simulink model "validation_gate_test"  (Simulink 7.6)
settings: Solver=FixedStepDiscrete  StartTime=0.0  StopTime=0  RelTol=1e-3
undefined symbols (not defined in the file or in its folder): Buoy_Count_Max, Buoy_Count_Min, Buoy_Max_Eccentricity, Buoy_Max_Extent, Buoy_Min_Eccentricity, Buoy_Min_Extent, Hedge_Hue, Iter_Segment_Thresh, Rec, SDTV, strel
libraries: vipconversions x6, vipgeotforms x3, simulink x2, viptextngfix x2, viptransforms x2, vipmorphops x1, vipanalysis x1
(part 1 of 2)
settings Model: Creator=Thing 1  LastModifiedBy=auvt

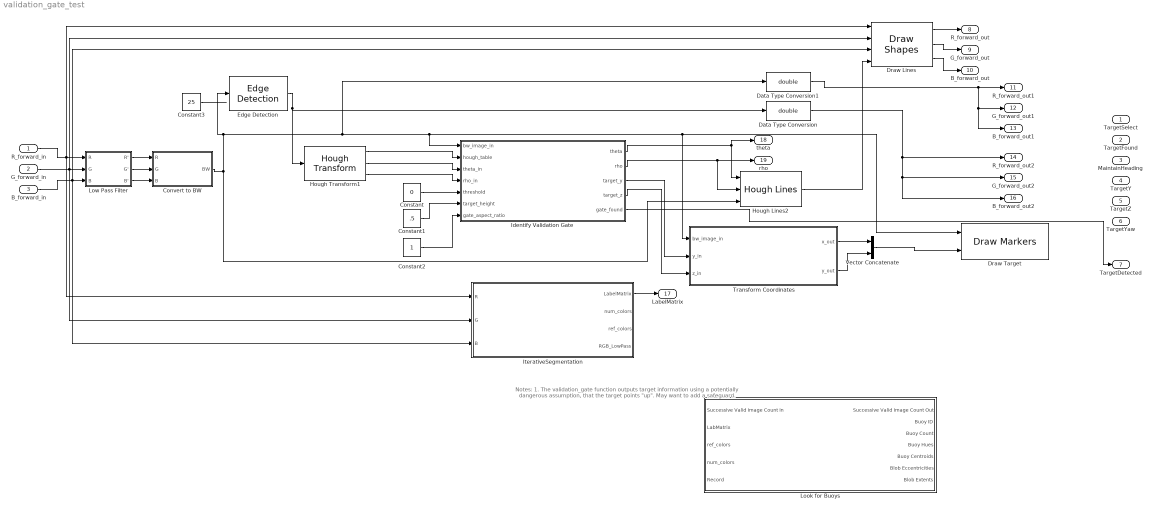
== system validation_gate_test ==
  note: Notes:
      | 1. The validation_gate function outputs target
      | information using a potentially dangerous
      | assumption, that the target points "up". May
      | want to add a safeguard.
  R_forward_in : Inport  PortDimensions=[120 160]
  G_forward_in : Inport  Port=2  PortDimensions=[120 160]
  B_forward_in : Inport  Port=3  PortDimensions=[120 160]
  Constant : Constant  Value=0  SampleTime=-1
  Constant1 : Constant  Value=.5  SampleTime=-1
  Constant2 : Constant  SampleTime=-1
  Constant3 : Constant  Value=25  SampleTime=-1
  Convert to BW : Subsystem
  Data Type Conversion : DataTypeConversion  OutDataTypeStr=double
  Data Type Conversion1 : DataTypeConversion  OutDataTypeStr=double
  Draw Lines : viptextngfix/Draw Shapes  DialogController=vipDDGCreate  DialogControllerArgs=DataTag3  shape=Lines  fill=off  fillClrSource=Specify via dialog  display=User-specified value  intensity=200  color=[.8 .8 .8]  opacity=0.6  viewport=Entire image  antialiasing=off  inType=Obsolete  imagePorts=Separate color signals  prodOutputMode=Binary point scaling  prodOutputWordLength=32  prodOutputFracLength=14  memoryMode=Specify word length  memoryWordLength=16  memoryFracLength=15  roundingMode=Floor  overflowMode=off
  Draw Target : viptextngfix/Draw Markers  DialogController=vipDDGCreate  DialogControllerArgs=DataTag4  shape=X-mark  size=7  fill=off  fillClrSource=Specify via dialog  display=User-specified value  intensity=200  color=0  opacity=0.6  viewport=Entire image  antialiasing=off  inType=Obsolete  imagePorts=One multidimensional signal  prodOutputMode=Binary point scaling  prodOutputWordLength=32  prodOutputFracLength=14  memoryMode=Specify word length  memoryWordLength=16  memoryFracLength=15  roundingMode=Floor  overflowMode=off
  Edge Detection : vipanalysis/Edge Detection  DialogController=vipDDGCreate  DialogControllerArgs=DataTag5  method=Sobel  outputType=Binary image  userDefinedThreshold=off  thresholdSource=Specify via dialog  threshold=20  thresholdTuning=3  edgeThinning=on  threshold_canny=[0.25 0.60]  autoPercent=70  sigma=1  roundingMode=Floor  overflowMode=off
  Hough Lines2 : viptransforms/Hough Lines  DialogController=vipDDGCreate  DialogControllerArgs=DataTag6  sineCompMethod=Trigonometric function  thetaRes=pi/180  firstCoeffMode=Specify word length  firstCoeffWordLength=16  firstCoeffFracLength=15  prodOutputMode=Binary point scaling  prodOutputWordLength=32  prodOutputFracLength=16  roundingMode=Nearest  overflowMode=on
  Hough Transform1 : viptransforms/Hough Transform  DialogController=vipDDGCreate  DialogControllerArgs=DataTag7  theta_res=.5*pi/180  rho_res=1  out_theta_rho=on  outdtmode=double  firstCoeffMode=Binary point scaling  firstCoeffWordLength=16  firstCoeffFracLength=14  secondCoeffMode=Binary point scaling  secondCoeffWordLength=32  secondCoeffFracLength=16  outputMode=Binary point scaling  outputWordLength=16  outputFracLength=0  accumMode=Binary point scaling  accumWordLength=32  accumFracLength=20  prodOutputMode=Binary point scaling  prodOutputWordLength=32  prodOutputFracLength=20  memoryMode=Binary point scaling  memoryWordLength=32  memoryFracLength=16  roundingMode=Nearest  overflowMode=on
  Identify Validation Gate : Stateflow chart  TreatAsAtomicUnit=on  SystemSampleTime=[1/30 0]
  IterativeSegmentation : Subsystem
      settings: UndoDeleteFcn=Stateflow.SLINSF.SimulinkMan.restorePreDeleteFcn  PreDeleteFcn=Stateflow.SLINSF.SimulinkMan.removePreDeleteFcn
  Look for Buoys : Subsystem
      settings: UndoDeleteFcn=Stateflow.SLINSF.SimulinkMan.restorePreDeleteFcn  PreDeleteFcn=Stateflow.SLINSF.SimulinkMan.removePreDeleteFcn
  Low Pass Filter : Subsystem
  Transform Coordinates : Stateflow chart  TreatAsAtomicUnit=on  SystemSampleTime=[1/30 0]
  Vector Concatenate : Concatenate  Mode=Multidimensional array
  TargetSelect : Outport  OutDataTypeStr=double
  TargetFound : Outport  Port=2  OutDataTypeStr=double
  MaintainHeading : Outport  Port=3  OutDataTypeStr=double
  TargetY : Outport  Port=4  OutDataTypeStr=double
  TargetZ : Outport  Port=5  OutDataTypeStr=double
  TargetYaw : Outport  Port=6  OutDataTypeStr=double
  TargetDetected : Outport  Port=7  OutDataTypeStr=double
  R_forward_out : Outport  Port=8  OutDataTypeStr=double
  G_forward_out : Outport  Port=9  OutDataTypeStr=double
  B_forward_out : Outport  Port=10  OutDataTypeStr=double
  R_forward_out1 : Outport  Port=11  OutDataTypeStr=double
  G_forward_out1 : Outport  Port=12  OutDataTypeStr=double
  B_forward_out1 : Outport  Port=13  OutDataTypeStr=double
  R_forward_out2 : Outport  Port=14  OutDataTypeStr=double
  G_forward_out2 : Outport  Port=15  OutDataTypeStr=double
  B_forward_out2 : Outport  Port=16  OutDataTypeStr=double
  LabelMatrix : Outport  Port=17  OutDataTypeStr=double
  theta : Outport  Port=18  OutDataTypeStr=double
  rho : Outport  Port=19  OutDataTypeStr=double
  wires:
  Convert to BW/1(BW) -> Hough Lines2/3, Edge Detection/1, Identify Validation Gate/1(bw_image_in), Transform Coordinates/1(bw_image_in), Draw Target/1, Data Type Conversion1/1
  Hough Transform1/1 -> Identify Validation Gate/2(hough_table)
  Hough Transform1/2 -> Identify Validation Gate/3(theta_in)
  Hough Transform1/3 -> Identify Validation Gate/4(rho_in)
  Edge Detection/1 -> Hough Transform1/1, Data Type Conversion/1
  Constant/1 -> Identify Validation Gate/5(threshold)
  Constant1/1 -> Identify Validation Gate/6(target_height)
  Constant2/1 -> Identify Validation Gate/7(gate_aspect_ratio)
  Identify Validation Gate/1(theta) -> Hough Lines2/1, theta/1
  Identify Validation Gate/2(rho) -> Hough Lines2/2, rho/1
  Identify Validation Gate/3(target_y) -> Transform Coordinates/2(y_in)
  Identify Validation Gate/4(target_z) -> Transform Coordinates/3(z_in)
  Transform Coordinates/1(x_out) -> Vector Concatenate/1
  Transform Coordinates/2(y_out) -> Vector Concatenate/2
  Vector Concatenate/1 -> Draw Target/2
  Identify Validation Gate/5(gate_found) -> TargetDetected/1
  Low Pass Filter/2(G') -> Convert to BW/2(G)
  Low Pass Filter/3(B') -> Convert to BW/3(B)
  G_forward_in/1 -> Low Pass Filter/2(G), IterativeSegmentation/2(G), Draw Lines/2
  B_forward_in/1 -> Low Pass Filter/3(B), IterativeSegmentation/3(B), Draw Lines/3
  Low Pass Filter/1(R') -> Convert to BW/1(R)
  R_forward_in/1 -> Low Pass Filter/1(R), IterativeSegmentation/1(R), Draw Lines/1
  Constant3/1 -> ?
  Data Type Conversion1/1 -> R_forward_out1/1, G_forward_out1/1, B_forward_out1/1
  IterativeSegmentation/1(LabelMatrix) -> LabelMatrix/1
  Data Type Conversion/1 -> R_forward_out2/1, G_forward_out2/1, B_forward_out2/1
  Draw Lines/1 -> R_forward_out/1
  Draw Lines/2 -> G_forward_out/1
  Draw Lines/3 -> B_forward_out/1
  Hough Lines2/1 -> Draw Lines/4

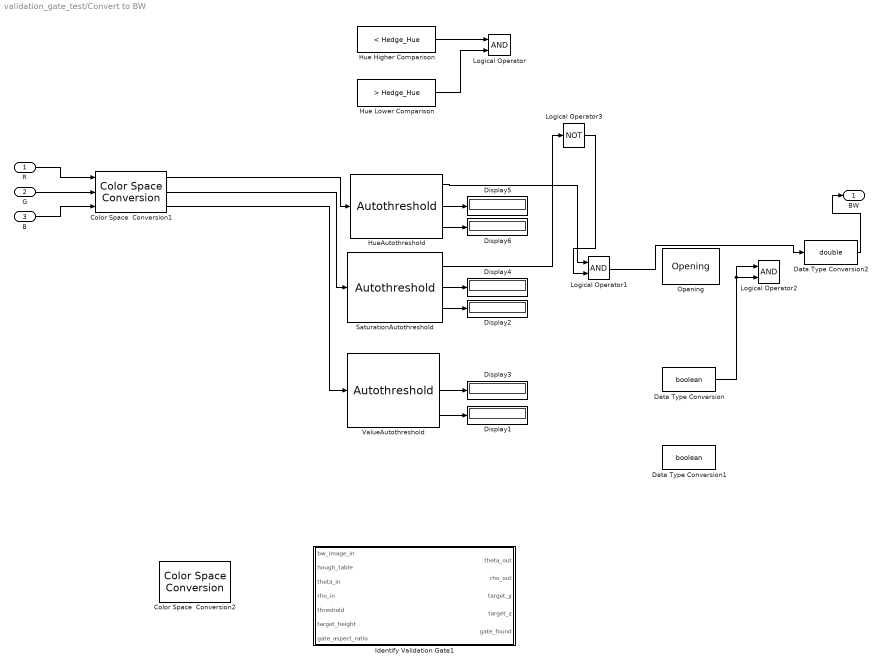
== system validation_gate_test/Convert to BW ==
  R : Inport  OutDataTypeStr=double
  G : Inport  Port=2  OutDataTypeStr=double
  B : Inport  Port=3  OutDataTypeStr=double
  Color Space  Conversion1 : vipconversions/Color Space  Conversion  conversion=Obsolete  conversionActive=R'G'B' to HSV  wp_str=D65  rec=Rec. 601 (SDTV)  sys=1125/60/2:1  imagePorts=Separate color signals
  Color Space  Conversion2 : vipconversions/Color Space  Conversion  conversion=Obsolete  conversionActive=R'G'B' to HSV  wp_str=D65  rec=Rec. 601 (SDTV)  sys=1125/60/2:1  imagePorts=Separate color signals
  Data Type Conversion : DataTypeConversion  OutDataTypeStr=boolean
  Data Type Conversion1 : DataTypeConversion  OutDataTypeStr=boolean
  Data Type Conversion2 : DataTypeConversion  OutDataTypeStr=double
  Display{1..6} (6 alike) : Display
  Hue Higher Comparison : simulink/Logic and Bit Operations/Compare To Constant  SystemSampleTime=-1  relop=<  const=Hedge_Hue  LogicOutDataTypeMode=boolean  ZeroCross=off
  Hue Lower Comparison : simulink/Logic and Bit Operations/Compare To Constant  SystemSampleTime=-1  relop=>  const=Hedge_Hue  LogicOutDataTypeMode=boolean  ZeroCross=off
  HueAutothreshold : vipconversions/Autothreshold  DialogController=vipDDGCreate  DialogControllerArgs=DataTag0  operator=>  threshOut=on  effMetricOut=on  userDefinedRange=off  umin=0  umax=255  outOfRngOpt=Warn and saturate  scaleThreshold=off  scaleFactor=1  P1Mode=Specify word length  P1WordLength=32  P1FracLength=30  P2Mode=Specify word length  P2WordLength=32  P2FracLength=22  P3Mode=Specify word length  P3WordLength=32  P3FracLength=14  P4Mode=Binary point scaling  P4WordLength=32  P4FracLength=15  Q1Mode=Specify word length  Q1WordLength=32  Q1FracLength=16  EMMode=Specify word length  EMWordLength=16  EMFracLength=14  roundingMode=Floor  overflowMode=off
  Identify Validation Gate1 : Stateflow chart  TreatAsAtomicUnit=on  SystemSampleTime=[1/30 0]
  Logical Operator : Logic  AllPortsSameDT=off  OutDataTypeStr=fixdt('boolean', 'DataTypeOverride', 'Off')
  Logical Operator1 : Logic
  Logical Operator2 : Logic
  Logical Operator3 : Logic  Operator=NOT
  Opening : vipmorphops/Opening  nhoodsrc=Specify via dialog  strel=strel('disk',2)
  SaturationAutothreshold : vipconversions/Autothreshold  DialogController=vipDDGCreate  DialogControllerArgs=DataTag1  operator=>  threshOut=on  effMetricOut=on  userDefinedRange=off  umin=0  umax=255  outOfRngOpt=Warn and saturate  scaleThreshold=off  scaleFactor=1  P1Mode=Specify word length  P1WordLength=32  P1FracLength=30  P2Mode=Specify word length  P2WordLength=32  P2FracLength=22  P3Mode=Specify word length  P3WordLength=32  P3FracLength=14  P4Mode=Binary point scaling  P4WordLength=32  P4FracLength=15  Q1Mode=Specify word length  Q1WordLength=32  Q1FracLength=16  EMMode=Specify word length  EMWordLength=16  EMFracLength=14  roundingMode=Floor  overflowMode=off
  ValueAutothreshold : vipconversions/Autothreshold  DialogController=vipDDGCreate  DialogControllerArgs=DataTag2  operator=>  threshOut=on  effMetricOut=on  userDefinedRange=off  umin=0  umax=255  outOfRngOpt=Warn and saturate  scaleThreshold=off  scaleFactor=1  P1Mode=Specify word length  P1WordLength=32  P1FracLength=30  P2Mode=Specify word length  P2WordLength=32  P2FracLength=22  P3Mode=Specify word length  P3WordLength=32  P3FracLength=14  P4Mode=Binary point scaling  P4WordLength=32  P4FracLength=15  Q1Mode=Specify word length  Q1WordLength=32  Q1FracLength=16  EMMode=Specify word length  EMWordLength=16  EMFracLength=14  roundingMode=Floor  overflowMode=off
  BW : Outport
  wires:
  Color Space  Conversion1/2 -> SaturationAutothreshold/1
  Color Space  Conversion1/1 -> HueAutothreshold/1
  SaturationAutothreshold/3 -> Display2/1
  ValueAutothreshold/2 -> Display3/1
  Color Space  Conversion1/3 -> ValueAutothreshold/1
  HueAutothreshold/2 -> Display5/1
  HueAutothreshold/3 -> Display6/1
  SaturationAutothreshold/2 -> Display4/1
  ValueAutothreshold/3 -> Display1/1
  Hue Higher Comparison/1 -> Logical Operator/1
  Hue Lower Comparison/1 -> Logical Operator/2
  Data Type Conversion/1 -> Logical Operator2/1, Logical Operator2/2
  R/1 -> Color Space  Conversion1/1
  G/1 -> Color Space  Conversion1/2
  B/1 -> Color Space  Conversion1/3
  Data Type Conversion2/1 -> BW/1
  Logical Operator1/1 -> Data Type Conversion2/1
  HueAutothreshold/1 -> Logical Operator1/1
  SaturationAutothreshold/1 -> Logical Operator3/1
  Logical Operator3/1 -> Logical Operator1/2

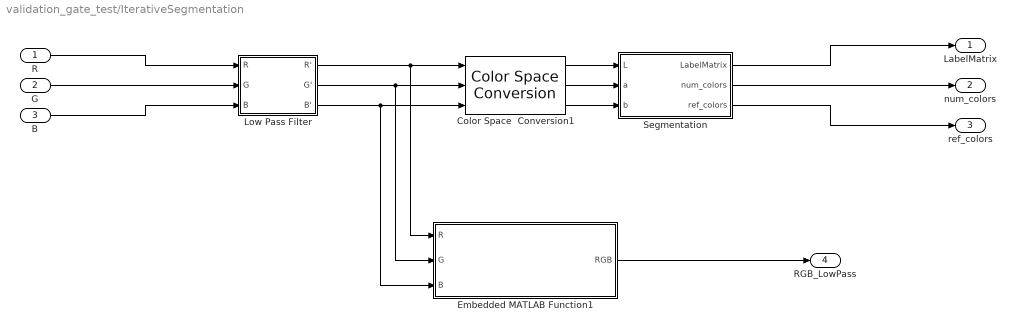
== system validation_gate_test/IterativeSegmentation ==
  R : Inport
  G : Inport  Port=2
  B : Inport  Port=3
  Color Space  Conversion1 : vipconversions/Color Space  Conversion  conversion=Obsolete  conversionActive=sR'G'B' to L*a*b*  wp_str=D50  rec=Rec. 601 (SDTV)  sys=1125/60/2:1  imagePorts=Separate color signals
  Embedded MATLAB Function1 : Stateflow chart  TreatAsAtomicUnit=on
  Low Pass Filter : Subsystem
  Segmentation : Subsystem
  LabelMatrix : Outport
  num_colors : Outport  Port=2
  ref_colors : Outport  Port=3
  RGB_LowPass : Outport  Port=4
  wires:
  Segmentation/3(ref_colors) -> ref_colors/1
  Segmentation/2(num_colors) -> num_colors/1
  Segmentation/1(LabelMatrix) -> LabelMatrix/1
  Low Pass Filter/3(B') -> Color Space  Conversion1/3, Embedded MATLAB Function1/3(B)
  Low Pass Filter/2(G') -> Color Space  Conversion1/2, Embedded MATLAB Function1/2(G)
  Low Pass Filter/1(R') -> Color Space  Conversion1/1, Embedded MATLAB Function1/1(R)
  Color Space  Conversion1/3 -> Segmentation/3(b)
  Color Space  Conversion1/2 -> Segmentation/2(a)
  Color Space  Conversion1/1 -> Segmentation/1(L)
  Embedded MATLAB Function1/1(RGB) -> RGB_LowPass/1
  R/1 -> Low Pass Filter/1(R)
  G/1 -> Low Pass Filter/2(G)
  B/1 -> Low Pass Filter/3(B)

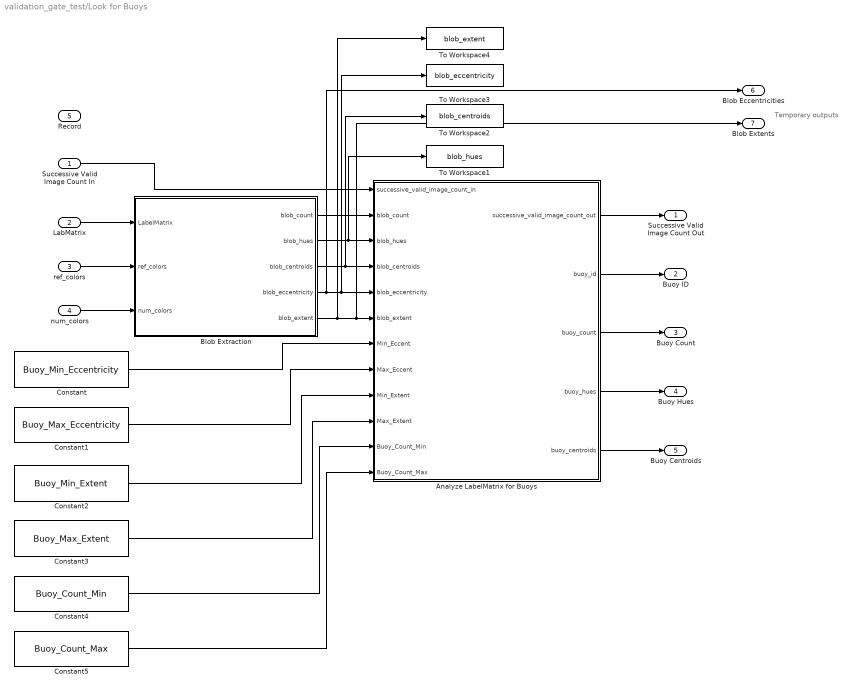
== system validation_gate_test/Look for Buoys ==
  note: Temporary outputs
  Successive Valid Image Count In : Inport
  LabMatrix : Inport  Port=2
  ref_colors : Inport  Port=3
  num_colors : Inport  Port=4
  Record : Inport  Port=5
  Analyze LabelMatrix for Buoys : Stateflow chart  TreatAsAtomicUnit=on
  Blob Extraction : Stateflow chart  TreatAsAtomicUnit=on
  Constant : Constant  Value=Buoy_Min_Eccentricity  SampleTime=-1
  Constant1 : Constant  Value=Buoy_Max_Eccentricity  SampleTime=-1
  Constant2 : Constant  Value=Buoy_Min_Extent  SampleTime=-1
  Constant3 : Constant  Value=Buoy_Max_Extent  SampleTime=-1
  Constant4 : Constant  Value=Buoy_Count_Min  SampleTime=-1
  Constant5 : Constant  Value=Buoy_Count_Max  SampleTime=-1
  To Workspace1 : ToWorkspace  VariableName=blob_hues  SampleTime=-1  SaveFormat=Array
  To Workspace2 : ToWorkspace  VariableName=blob_centroids  SampleTime=-1  SaveFormat=Array
  To Workspace3 : ToWorkspace  VariableName=blob_eccentricity  SampleTime=-1  SaveFormat=Array
  To Workspace4 : ToWorkspace  VariableName=blob_extent  SampleTime=-1  SaveFormat=Array
  Successive Valid Image Count Out : Outport
  Buoy ID : Outport  Port=2
  Buoy Count : Outport  Port=3
  Buoy Hues : Outport  Port=4
  Buoy Centroids : Outport  Port=5
  Blob Eccentricities : Outport  Port=6
  Blob Extents : Outport  Port=7
  wires:
  num_colors/1 -> Blob Extraction/3(num_colors)
  LabMatrix/1 -> Blob Extraction/1(LabelMatrix)
  Blob Extraction/1(blob_count) -> Analyze LabelMatrix for Buoys/2(blob_count)
  Blob Extraction/2(blob_hues) -> Analyze LabelMatrix for Buoys/3(blob_hues), To Workspace1/1
  Blob Extraction/3(blob_centroids) -> Analyze LabelMatrix for Buoys/4(blob_centroids), To Workspace2/1
  Blob Extraction/4(blob_eccentricity) -> Analyze LabelMatrix for Buoys/5(blob_eccentricity), To Workspace3/1, Blob Eccentricities/1
  Blob Extraction/5(blob_extent) -> To Workspace4/1, Analyze LabelMatrix for Buoys/6(blob_extent), Blob Extents/1
  Constant/1 -> Analyze LabelMatrix for Buoys/7(Min_Eccent)
  Constant1/1 -> Analyze LabelMatrix for Buoys/8(Max_Eccent)
  Constant2/1 -> Analyze LabelMatrix for Buoys/9(Min_Extent)
  Constant3/1 -> Analyze LabelMatrix for Buoys/10(Max_Extent)
  Constant4/1 -> Analyze LabelMatrix for Buoys/11(Buoy_Count_Min)
  Constant5/1 -> Analyze LabelMatrix for Buoys/12(Buoy_Count_Max)
  Analyze LabelMatrix for Buoys/1(successive_valid_image_count_out) -> Successive Valid Image Count Out/1
  Analyze LabelMatrix for Buoys/3(buoy_count) -> Buoy Count/1
  Analyze LabelMatrix for Buoys/4(buoy_hues) -> Buoy Hues/1
  Analyze LabelMatrix for Buoys/5(buoy_centroids) -> Buoy Centroids/1
  Successive Valid Image Count In/1 -> Analyze LabelMatrix for Buoys/1(successive_valid_image_count_in)
  ref_colors/1 -> Blob Extraction/2(ref_colors)
  Analyze LabelMatrix for Buoys/2(buoy_id) -> Buoy ID/1

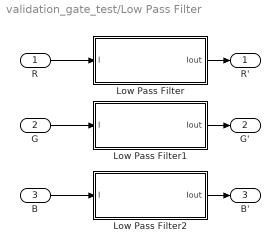
== system validation_gate_test/Low Pass Filter ==
  R : Inport
  G : Inport  Port=2
  B : Inport  Port=3
  Low Pass Filter : Stateflow chart  TreatAsAtomicUnit=on
  Low Pass Filter1 : Stateflow chart  TreatAsAtomicUnit=on
  Low Pass Filter2 : Stateflow chart  TreatAsAtomicUnit=on
  R' : Outport
  G' : Outport  Port=2
  B' : Outport  Port=3
  wires:
  Low Pass Filter/1(Iout) -> R'/1
  Low Pass Filter2/1(Iout) -> B'/1
  Low Pass Filter1/1(Iout) -> G'/1
  B/1 -> Low Pass Filter2/1(I)
  G/1 -> Low Pass Filter1/1(I)
  R/1 -> Low Pass Filter/1(I)

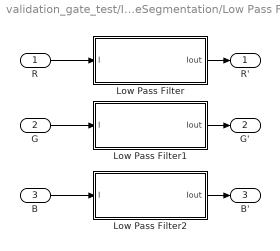
== system validation_gate_test/IterativeSegmentation/Low Pass Filter ==
  R : Inport
  G : Inport  Port=2
  B : Inport  Port=3
  Low Pass Filter : Stateflow chart  TreatAsAtomicUnit=on
  Low Pass Filter1 : Stateflow chart  TreatAsAtomicUnit=on
  Low Pass Filter2 : Stateflow chart  TreatAsAtomicUnit=on
  R' : Outport
  G' : Outport  Port=2
  B' : Outport  Port=3
  wires:
  Low Pass Filter/1(Iout) -> R'/1
  Low Pass Filter2/1(Iout) -> B'/1
  Low Pass Filter1/1(Iout) -> G'/1
  B/1 -> Low Pass Filter2/1(I)
  G/1 -> Low Pass Filter1/1(I)
  R/1 -> Low Pass Filter/1(I)

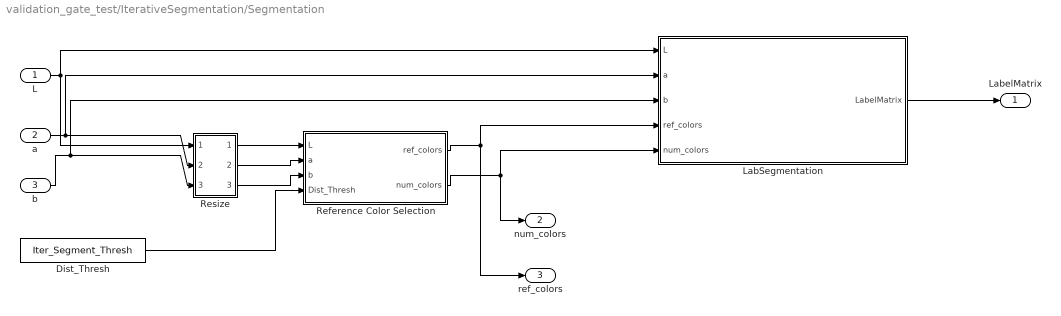
== system validation_gate_test/IterativeSegmentation/Segmentation ==
  L : Inport
  a : Inport  Port=2
  b : Inport  Port=3
  Dist_Thresh : Constant  Value=Iter_Segment_Thresh  SampleTime=-1
  LabSegmentation : Stateflow chart  TreatAsAtomicUnit=on
  Reference Color Selection : Stateflow chart  TreatAsAtomicUnit=on
  Resize : Subsystem
  LabelMatrix : Outport
  num_colors : Outport  Port=2
  ref_colors : Outport  Port=3
  wires:
  Dist_Thresh/1 -> Reference Color Selection/4(Dist_Thresh)
  LabSegmentation/1(LabelMatrix) -> LabelMatrix/1
  Reference Color Selection/2(num_colors) -> LabSegmentation/5(num_colors), num_colors/1
  Reference Color Selection/1(ref_colors) -> ref_colors/1, LabSegmentation/4(ref_colors)
  Resize/3(Out3) -> Reference Color Selection/3(b)
  Resize/2(Out2) -> Reference Color Selection/2(a)
  Resize/1(Out1) -> Reference Color Selection/1(L)
  b/1 -> LabSegmentation/3(b), Resize/3(In3)
  a/1 -> LabSegmentation/2(a), Resize/2(In2)
  L/1 -> LabSegmentation/1(L), Resize/1(In1)

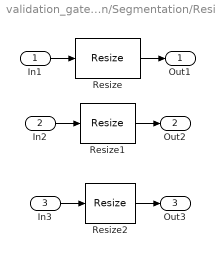
== system validation_gate_test/IterativeSegmentation/Segmentation/Resize ==
  In1 : Inport
  In2 : Inport  Port=2
  In3 : Inport  Port=3
  Resize : vipgeotforms/Resize  DialogController=vipDDGCreate  DialogControllerArgs=DataTag8  specify=Number of output rows and columns  rfactor=[]  outCols=25  outRows=25  outRowsCols=[60 80]  interp_method=Bilinear  antialias=on  useROI=off  roiFlag=off  prodOutputMode=Binary point scaling  prodOutputWordLength=32  prodOutputFracLength=10  roundingMode=Nearest  overflowMode=on
  Resize1 : vipgeotforms/Resize  DialogController=vipDDGCreate  DialogControllerArgs=DataTag9  specify=Number of output rows and columns  rfactor=[200 150]  outCols=25  outRows=25  outRowsCols=[60 80]  interp_method=Bilinear  antialias=on  useROI=off  roiFlag=off  prodOutputMode=Binary point scaling  prodOutputWordLength=32  prodOutputFracLength=10  roundingMode=Nearest  overflowMode=on
  Resize2 : vipgeotforms/Resize  DialogController=vipDDGCreate  DialogControllerArgs=DataTag10  specify=Number of output rows and columns  rfactor=[200 150]  outCols=25  outRows=25  outRowsCols=[60 80]  interp_method=Bilinear  antialias=on  useROI=off  roiFlag=off  prodOutputMode=Binary point scaling  prodOutputWordLength=32  prodOutputFracLength=10  roundingMode=Nearest  overflowMode=on
  Out1 : Outport
  Out2 : Outport  Port=2
  Out3 : Outport  Port=3
  wires:
  Resize2/1 -> Out3/1
  In3/1 -> Resize2/1
  Resize1/1 -> Out2/1
  In2/1 -> Resize1/1
  Resize/1 -> Out1/1
  In1/1 -> Resize/1

== matlab function Identify Validation Gate ==
  data: bw_image_in input double; hough_table input double; theta output double; rho output double; target_y output double; target_z output double; gate_found output double; theta_in input double; rho_in input double; threshold input double; target_height input double; gate_aspect_ratio input double
function [theta, rho, target_y, target_z, gate_found] = validation_gate(bw_image_in, hough_table, theta_in, rho_in, threshold, target_height, gate_aspect_ratio)
%#eml

% This function attempts to identfiy the validation gate, and returns line
%   information, targeting information, and a true/false gate_found
%   parameter.
%
% 5-29-11
%
% Input
%
%   target_height = fraction of goal post height to aim AUV at
%   gate_aspect_ratio = used to infer unknown points with little extra
%     processing (height/width of large T-shape)
%
% Output
%
% Notes:
%   The hough_table is destroyed in this function (acceptable if
%     hough_table is not an output)
%   Process:
%     1. Identify primary, relatively "long" lines
%     2. 

% Initialize
peak_tol_ratio = .1;  % Fraction of max(rows,cols) of image within which a
%                         peak is assumed to reside; this helps reduce
%                         incorrect line extraction
max_num_lines = 150;  % Considers this many popular lines as candidates

[rho_length, theta_length] = size(hough_table);
[rows, cols] = size(bw_image_in);
rho_tol = .1*max(rows,cols);
theta_tol = 10*pi/180;  % Tolerence within which two slopes are equal (radians)

rho_out = zeros(1,3);
theta_out = zeros(1,3);
rho = zeros(1,max_num_lines);
theta = zeros(1,max_num_lines);

% Theta and rho resolutions for this function only; used to filter lines
%   that are not within eps_rho, eps_theta
eps_rho = 10;
eps_theta = 5*pi/180;



% Apply appropriate threshold
hough_table = hough_table.*( hough_table > threshold );


% Identify the most likely max_num_lines lines
i_index = ones(1,max_num_lines);
j_index = ones(1,max_num_lines);

m = 1;
while( m <= max_num_lines )
    
    max_votes = 0;
    for i = 1:rho_length
        for j = 1:theta_length
            if( hough_table(i,j) > max_votes )
                i_index(m) = i;
                j_index(m) = j;
                max_votes = hough_table(i,j);
            end
        end
    end
    
    rho(m) = rho_in(i_index(m));
    theta(m) = theta_in(j_index(m));
    hough_table(i_index(m),j_index(m)) = 0;
    m = m + 1;
    
end


% Extract the three most popular lines that fit the geometric criteria for
%   the goalpost
rho_out(1) = rho(1);
theta_out(1) = theta(1);

m = 2;

%rho_radius = 10;
%theta_radius = 5*pi/180;

for i = 2:max_num_lines
    
    % If rho, theta indicate that the line is either "horizontal" or
    %   "vertical", then store as a possible validation gate line
    if( abs( theta(m) - pi/2 ) <= eps_theta || abs( theta(m) + pi/2 ) <= eps_theta )
    
%    % If rho, theta do not match within tolerance, then store as the next
%    %   line
%%    if( ( (rho(m) - rho(1))/rho_radius)^2 + ( (theta(m) - theta(1))/theta_radius)^2 > 1 )
%%    if( abs(rho(i) - rho(i-1)) >= 30 )
        rho_out(m) = rho(i);
        theta_out(m) = theta(i);
        m = m + 1;
        if( m > 3 )
            break;
        end
    end
    
end


% Determine whether or not the top three lines constitute the goal post
%   Note that the Simulink block feeding this function keeps theta between
%   +/- pi/2
if( abs(theta_out(1) - theta_out(2)) < theta_tol && ( max(theta_out(1),theta_out(3)) - min(theta_out(1),theta_out(3)) - pi/2 < theta_tol ) )
    gate_found = 1;
    avg_slope = -( 1/tan(theta_out(1)) + 1/tan(theta_out(2)) )/2;
    y1 = ( (rho_out(1)/cos(theta_out(1))) - (rho_out(3)/cos(theta_out(3))) )*( 1/( tan(theta_out(1)) - tan(theta_out(3)) ) );
    x1 = ( 1/cos(theta_out(1)) )*( rho_out(1) - y1*sin(theta_out(1)) );
    y2 = ( (rho_out(2)/cos(theta_out(2))) - (rho_out(3)/cos(theta_out(3))) )*( 1/( tan(theta_out(2)) - tan(theta_out(3)) ) );
    x2 = ( 1/cos(theta_out(2)) )*( rho_out(2) - y2*sin(theta_out(2)) );
    
elseif( abs(theta_out(1) - theta_out(3)) < theta_tol && ( max(theta_out(1),theta_out(2)) - min(theta_out(1),theta_out(2)) - pi/2 < theta_tol ) )
    gate_found = 1;
    avg_slope = -( 1/tan(theta_out(1)) + 1/tan(theta_out(3)) )/2;
    y1 = ( (rho_out(1)/cos(theta_out(1))) - (rho_out(2)/cos(theta_out(2))) )*( 1/( tan(theta_out(1)) - tan(theta_out(2)) ) );
    x1 = ( 1/cos(theta_out(1)) )*( rho_out(1) - y1*sin(theta_out(1)) );
    y2 = ( (rho_out(2)/cos(theta_out(2))) - (rho_out(3)/cos(theta_out(3))) )*( 1/( tan(theta_out(2)) - tan(theta_out(3)) ) );
    x2 = ( 1/cos(theta_out(2)) )*( rho_out(2) - y2*sin(theta_out(2)) );
    
elseif( abs(theta_out(2) - theta_out(3)) < theta_tol && ( max(theta_out(1),theta_out(2)) - min(theta_out(1),theta_out(2)) - pi/2 < theta_tol ) )
    gate_found = 1;
    avg_slope = -( 1/tan(theta_out(2)) + 1/tan(theta_out(3)) )/2;
    y1 = ( (rho_out(1)/cos(theta_out(1))) - (rho_out(2)/cos(theta_out(2))) )*( 1/( tan(theta_out(1)) - tan(theta_out(2)) ) );
    x1 = ( 1/cos(theta_out(1)) )*( rho_out(1) - y1*sin(theta_out(1)) );
    y2 = ( (rho_out(1)/cos(theta_out(1))) - (rho_out(3)/cos(theta_out(3))) )*( 1/( tan(theta_out(1)) - tan(theta_out(3)) ) );
    x2 = ( 1/cos(theta_out(1)) )*( rho_out(1) - y2*sin(theta_out(1)) );
    
else
    gate_found = 0;
    avg_slope = 0;
    
    x1 = 0;
    y1 = 0;
    x2 = 0;
    y2 = 0;
    
end


% Determine targeting information (default to center of viewing area if no
%   gate found)
if( gate_found ~= 0 )
    
    % Determine width and half-height (to center of goal post)
    w = sqrt( (x2 - x1)^2 + (y2 - y1)^2 );
    hh = target_height*gate_aspect_ratio*w;
    
    % Project a line "up" (relative to camera) and determine target
    %   information
    x12 = (x1 + x2)/2;
    y12 = (y1 + y2)/2;
    
    u = [1 -abs(avg_slope)];
    u = u./norm(u);
    
    target_x = x12 + hh*u(1);
    target_y = y12 + hh*u(2);
    
    
    % old code that works, partially
    %phi = atan(avg_slope);
    %target_x = x12 - hh*cos(phi);
    %target_y = y12 - hh*sin(phi);
    
    
    
    
    
    
    %{
    intercept = y12 - avg_slope*x12;
    
    a = avg_slope^2 + 1;
    b = 2*(avg_slope*(intercept - y12) - x12);
    c = x12^2 + (avg_slope - y12)^2 - hh^2;
    
    target_x = real( (-b + sqrt(b^2 - 4*a*c))/(2*a) );
    target_y = avg_slope*target_x + intercept;
    %}
    
    
    
    % Transform target x, y to global coordinate system
    target_z = target_y - floor(rows/2);
    target_y = target_x - floor(cols/2);
    
else
    
    % Default is center of viewing area
    target_x = 0;
    target_y = 0;
    target_z = 0;
    
end


return

== matlab function Transform Coordinates ==
  data: bw_image_in input double; y_in input double; x_out output double; y_out output double; z_in input double
function [x_out, y_out] = transform_G2L(bw_image_in, y_in, z_in)
% This function, "transform Global to Local coordinates," simply transforms
%   global coordinates that are sent to the controller into local
%   coordinates that can be displayed over images.
%
% 5-29-11

[rows, cols] = size(bw_image_in);
x_out = z_in + floor(rows/2);
y_out = y_in + floor(cols/2);

return

== matlab function Convert to BW/Identify Validation Gate1 ==
  data: bw_image_in input double; hough_table input double; theta_out output double; rho_out output double; target_y output double; target_z output double; gate_found output double; theta_in input double; rho_in input double; threshold input double; target_height input double; gate_aspect_ratio input double
function [theta_out, rho_out, target_y, target_z, gate_found] = hue_filter(bw_image_in, hough_table, theta_in, rho_in, threshold, target_height, gate_aspect_ratio)
%#eml

% This function attempts to identfiy the validation gate, and returns line
%   information, targeting information, and a true/false gate_found
%   parameter.
%
% 5-29-11
%
% Input
%
%   target_height = fraction of goal post height to aim AUV at
%   gate_aspect_ratio = used to infer unknown points with little extra
%     processing (height/width of large T-shape)
%
% Output
%
% Notes:
%   The hough_table is destroyed in this function (acceptable if
%     hough_table is not an output)
%   Process:
%     1. Identify primary, relatively "long" lines
%     2. 

% Initialize
peak_tol_ratio = .1;  % Fraction of max(rows,cols) of image within which a
%                         peak is assumed to reside; this helps reduce
%                         incorrect line extraction
max_num_lines = 10;  % Considers this many popular lines as candidates

[rho_length, theta_length] = size(hough_table);
[rows, cols] = size(bw_image_in);
rho_tol = .1*max(rows,cols);
theta_tol = 10*pi/180;  % Tolerence within which two slopes are equal (radians)

rho_out = zeros(1,3);
theta_out = zeros(1,3);
rho = zeros(1,max_num_lines);
theta = zeros(1,max_num_lines);



% Apply appropriate threshold
hough_table = hough_table.*( hough_table > threshold );


% Identify the most likely max_num_lines lines
i_index = ones(1,max_num_lines);
j_index = ones(1,max_num_lines);

m = 1;
while( m <= max_num_lines )
    
    max_votes = 0;
    for i = 1:rho_length
        for j = 1:theta_length
            if( hough_table(i,j) > max_votes )
                i_index(m) = i;
                j_index(m) = j;
                max_votes = hough_table(i,j);
            end
        end
    end
    
    rho(m) = rho_in(i_index(m));
    theta(m) = theta_in(j_index(m));
    hough_table(i_index(m),j_index(m)) = 0;
    m = m + 1;
    
end


% Extract the three most popular lines that fit the geometric criteria for
%   the goalpost
rho_out(1) = rho(1);
theta_out(1) = theta(1);

m = 2;

%rho_radius = 10;
%theta_radius = 5*pi/180;

for i = 2:max_num_lines
    
    % If rho, theta do not match within tolerance, then store as the next
    %   line
%    if( ( (rho(m) - rho(1))/rho_radius)^2 + ( (theta(m) - theta(1))/theta_radius)^2 > 1 )
    if( abs(rho(i) - rho(i-1)) >= 30 )
        rho_out(m) = rho(i);
        theta_out(m) = theta(i);
        m = m + 1;
        if( m > 3 )
            break;
        end
    end
    
end


% Determine whether or not the top three lines constitute the goal post
%   Note that the Simulink block feeding this function keeps theta between
%   +/- pi/2
if( abs(theta_out(1) - theta_out(2)) < theta_tol && ( max(theta_out(1),theta_out(3)) - min(theta_out(1),theta_out(3)) - pi/2 < theta_tol ) )
    gate_found = 1;
    avg_slope = -( 1/tan(theta_out(1)) + 1/tan(theta_out(2)) )/2;
    y1 = ( (rho_out(1)/cos(theta_out(1))) - (rho_out(3)/cos(theta_out(3))) )*( 1/( tan(theta_out(1)) - tan(theta_out(3)) ) );
    x1 = ( 1/cos(theta_out(1)) )*( rho_out(1) - y1*sin(theta_out(1)) );
    y2 = ( (rho_out(2)/cos(theta_out(2))) - (rho_out(3)/cos(theta_out(3))) )*( 1/( tan(theta_out(2)) - tan(theta_out(3)) ) );
    x2 = ( 1/cos(theta_out(2)) )*( rho_out(2) - y2*sin(theta_out(2)) );
    
elseif( abs(theta_out(1) - theta_out(3)) < theta_tol && ( max(theta_out(1),theta_out(2)) - min(theta_out(1),theta_out(2)) - pi/2 < theta_tol ) )
    gate_found = 1;
    avg_slope = -( 1/tan(theta_out(1)) + 1/tan(theta_out(3)) )/2;
    y1 = ( (rho_out(1)/cos(theta_out(1))) - (rho_out(2)/cos(theta_out(2))) )*( 1/( tan(theta_out(1)) - tan(theta_out(2)) ) );
    x1 = ( 1/cos(theta_out(1)) )*( rho_out(1) - y1*sin(theta_out(1)) );
    y2 = ( (rho_out(2)/cos(theta_out(2))) - (rho_out(3)/cos(theta_out(3))) )*( 1/( tan(theta_out(2)) - tan(theta_out(3)) ) );
    x2 = ( 1/cos(theta_out(2)) )*( rho_out(2) - y2*sin(theta_out(2)) );
    
elseif( abs(theta_out(2) - theta_out(3)) < theta_tol && ( max(theta_out(1),theta_out(2)) - min(theta_out(1),theta_out(2)) - pi/2 < theta_tol ) )
    gate_found = 1;
    avg_slope = -( 1/tan(theta_out(2)) + 1/tan(theta_out(3)) )/2;
    y1 = ( (rho_out(1)/cos(theta_out(1))) - (rho_out(2)/cos(theta_out(2))) )*( 1/( tan(theta_out(1)) - tan(theta_out(2)) ) );
    x1 = ( 1/cos(theta_out(1)) )*( rho_out(1) - y1*sin(theta_out(1)) );
    y2 = ( (rho_out(1)/cos(theta_out(1))) - (rho_out(3)/cos(theta_out(3))) )*( 1/( tan(theta_out(1)) - tan(theta_out(3)) ) );
    x2 = ( 1/cos(theta_out(1)) )*( rho_out(1) - y2*sin(theta_out(1)) );
    
else
    gate_found = 0;
    avg_slope = 0;
    
    x1 = 0;
    y1 = 0;
    x2 = 0;
    y2 = 0;
    
end


% Determine targeting information (default to center of viewing area if no
%   gate found)
if( gate_found ~= 0 )
    
    % Determine width and half-height (to center of goal post)
    w = sqrt( (x2 - x1)^2 + (y2 - y1)^2 );
    hh = target_height*gate_aspect_ratio*w;
    
    % Project a line "up" (relative to camera) and determine target
    %   information
    x12 = (x1 + x2)/2;
    y12 = (y1 + y2)/2;
    
    u = [1 -abs(avg_slope)];
    u = u./norm(u);
    
    target_x = x12 + hh*u(1);
    target_y = y12 + hh*u(2);
    
    
    % old code that works, partially
    %phi = atan(avg_slope);
    %target_x = x12 - hh*cos(phi);
    %target_y = y12 - hh*sin(phi);
    
    
    
    
    
    
    %{
    intercept = y12 - avg_slope*x12;
    
    a = avg_slope^2 + 1;
    b = 2*(avg_slope*(intercept - y12) - x12);
    c = x12^2 + (avg_slope - y12)^2 - hh^2;
    
    target_x = real( (-b + sqrt(b^2 - 4*a*c))/(2*a) );
    target_y = avg_slope*target_x + intercept;
    %}
    
    
    
    % Transform target x, y to global coordinate system
    target_z = target_y - floor(rows/2);
    target_y = target_x - floor(cols/2);
    
else
    
    % Default is center of viewing area
    target_x = 0;
    target_y = 0;
    target_z = 0;
    
end


return

== matlab function IterativeSegmentation/Low Pass Filter/Low Pass Filter ==
  data: I input double; Iout output double
function Iout = GaussianBlurr(I)
% This function calculates the gaussian blur of an intensity image

sigma = sqrt(2);

Grows = 3;    % Gaussian matrix rows
Gcols = 3;    % Gaussian matrix columns

[Irows Icols] = size(I);

Iout = double(zeros(Irows,Icols));

Trows = Irows - Grows + 1;
Tcols = Icols - Gcols + 1;
Itemp = double(zeros(Trows,Tcols));

G = zeros(Grows,Gcols);

FirstRow = ceil(-Grows/2);
LastRow = floor(Grows/2);
FirstCol = ceil(-Gcols/2);
LastCol = floor(Gcols/2);
Gsum = 0;
for i=FirstRow:LastRow
    for j = FirstCol:LastCol
        G(i-FirstRow+1,j-FirstCol+1) = exp(-(j*j+i*i)/(2*sigma*sigma));
        Gsum = Gsum + G(i-FirstRow+1,j-FirstCol+1);
    end
end

G = G./Gsum;

Itemp = conv2(double(I),double(G),'valid');

% reflect boundaries to keep image the same size
% top
Iout((1:LastRow),(LastCol+1:Icols-LastCol)) = Itemp((1:LastRow),(1:Tcols));
% bottom
Iout((Irows-LastRow+1:Irows),(LastCol+1:Icols-LastCol)) = Itemp((Trows-LastRow+1:Trows),(1:Tcols));
% left
Iout((1+LastRow:Irows-LastRow),(1:LastCol)) = Itemp((1:Trows),(1:LastCol));
% right
Iout((1+LastRow:Irows-LastRow),(Icols-LastCol+1:Icols)) = Itemp((1:Trows),(Tcols-LastCol+1:Tcols));
% center
Iout((1+LastRow:Irows-LastRow),(1+LastCol:Icols-LastCol)) = Itemp;
% top left corner
Iout(1:LastRow,1:LastCol) = Itemp(1:LastRow,1:LastCol);
% top right corner
Iout(1:LastRow,Icols-LastCol:Icols) = Itemp(1:LastRow,Tcols-LastCol:Tcols);
% bottom left corner
Iout(Irows-LastRow:Irows,1:LastCol) = Itemp(Trows-LastRow:Trows,1:LastCol);
% bottom right corner
Iout(Irows-LastRow:Irows,Icols-LastCol:Icols) = Itemp(Trows-LastRow:Trows,Tcols-LastCol:Tcols);

return

== matlab function IterativeSegmentation/Low Pass Filter/Low Pass Filter1 ==
  data: I input double; Iout output double
function Iout = GaussianBlurr(I)
% This function calculates the gaussian blur of an intensity image

sigma = sqrt(2);

Grows = 3;    % Gaussian matrix rows
Gcols = 3;    % Gaussian matrix columns

[Irows Icols] = size(I);

Iout = double(zeros(Irows,Icols));

Trows = Irows - Grows + 1;
Tcols = Icols - Gcols + 1;
Itemp = double(zeros(Trows,Tcols));

G = zeros(Grows,Gcols);

FirstRow = ceil(-Grows/2);
LastRow = floor(Grows/2);
FirstCol = ceil(-Gcols/2);
LastCol = floor(Gcols/2);
Gsum = 0;
for i=FirstRow:LastRow
    for j = FirstCol:LastCol
        G(i-FirstRow+1,j-FirstCol+1) = exp(-(j*j+i*i)/(2*sigma*sigma));
        Gsum = Gsum + G(i-FirstRow+1,j-FirstCol+1);
    end
end

G = G./Gsum;

Itemp = conv2(double(I),double(G),'valid');

% reflect boundaries to keep image the same size
% top
Iout((1:LastRow),(LastCol+1:Icols-LastCol)) = Itemp((1:LastRow),(1:Tcols));
% bottom
Iout((Irows-LastRow+1:Irows),(LastCol+1:Icols-LastCol)) = Itemp((Trows-LastRow+1:Trows),(1:Tcols));
% left
Iout((1+LastRow:Irows-LastRow),(1:LastCol)) = Itemp((1:Trows),(1:LastCol));
% right
Iout((1+LastRow:Irows-LastRow),(Icols-LastCol+1:Icols)) = Itemp((1:Trows),(Tcols-LastCol+1:Tcols));
% center
Iout((1+LastRow:Irows-LastRow),(1+LastCol:Icols-LastCol)) = Itemp;
% top left corner
Iout(1:LastRow,1:LastCol) = Itemp(1:LastRow,1:LastCol);
% top right corner
Iout(1:LastRow,Icols-LastCol:Icols) = Itemp(1:LastRow,Tcols-LastCol:Tcols);
% bottom left corner
Iout(Irows-LastRow:Irows,1:LastCol) = Itemp(Trows-LastRow:Trows,1:LastCol);
% bottom right corner
Iout(Irows-LastRow:Irows,Icols-LastCol:Icols) = Itemp(Trows-LastRow:Trows,Tcols-LastCol:Tcols);

return

== matlab function IterativeSegmentation/Low Pass Filter/Low Pass Filter2 ==
  data: I input double; Iout output double
function Iout = GaussianBlurr(I)
% This function calculates the gaussian blur of an intensity image

sigma = sqrt(2);

Grows = 3;    % Gaussian matrix rows
Gcols = 3;    % Gaussian matrix columns

[Irows Icols] = size(I);

Iout = double(zeros(Irows,Icols));

Trows = Irows - Grows + 1;
Tcols = Icols - Gcols + 1;
Itemp = double(zeros(Trows,Tcols));

G = zeros(Grows,Gcols);

FirstRow = ceil(-Grows/2);
LastRow = floor(Grows/2);
FirstCol = ceil(-Gcols/2);
LastCol = floor(Gcols/2);
Gsum = 0;
for i=FirstRow:LastRow
    for j = FirstCol:LastCol
        G(i-FirstRow+1,j-FirstCol+1) = exp(-(j*j+i*i)/(2*sigma*sigma));
        Gsum = Gsum + G(i-FirstRow+1,j-FirstCol+1);
    end
end

G = G./Gsum;

Itemp = conv2(double(I),double(G),'valid');

% reflect boundaries to keep image the same size
% top
Iout((1:LastRow),(LastCol+1:Icols-LastCol)) = Itemp((1:LastRow),(1:Tcols));
% bottom
Iout((Irows-LastRow+1:Irows),(LastCol+1:Icols-LastCol)) = Itemp((Trows-LastRow+1:Trows),(1:Tcols));
% left
Iout((1+LastRow:Irows-LastRow),(1:LastCol)) = Itemp((1:Trows),(1:LastCol));
% right
Iout((1+LastRow:Irows-LastRow),(Icols-LastCol+1:Icols)) = Itemp((1:Trows),(Tcols-LastCol+1:Tcols));
% center
Iout((1+LastRow:Irows-LastRow),(1+LastCol:Icols-LastCol)) = Itemp;
% top left corner
Iout(1:LastRow,1:LastCol) = Itemp(1:LastRow,1:LastCol);
% top right corner
Iout(1:LastRow,Icols-LastCol:Icols) = Itemp(1:LastRow,Tcols-LastCol:Tcols);
% bottom left corner
Iout(Irows-LastRow:Irows,1:LastCol) = Itemp(Trows-LastRow:Trows,1:LastCol);
% bottom right corner
Iout(Irows-LastRow:Irows,Icols-LastCol:Icols) = Itemp(Trows-LastRow:Trows,Tcols-LastCol:Tcols);

return

== matlab function Look for Buoys/Analyze LabelMatrix for Buoys ==
  data: successive_valid_image_count_in input double; successive_valid_image_count_out output double; buoy_id output double; blob_count input double; blob_hues input double; blob_centroids input double; buoy_count output double; buoy_hues output double; buoy_centroids output double; blob_eccentricity input double; blob_extent input double; Min_Eccent input double; Max_Eccent input double; Min_Extent input double; Max_Extent input double; Buoy_Count_Min input double; Buoy_Count_Max input double
function [successive_valid_image_count_out, buoy_id, buoy_count, buoy_hues, buoy_centroids] = Buoy_Extraction(successive_valid_image_count_in, blob_count, blob_hues, blob_centroids, blob_eccentricity, blob_extent, Min_Eccent, Max_Eccent, Min_Extent, Max_Extent, Buoy_Count_Min, Buoy_Count_Max)
% This function takes in vectors representing blobs present in the image,
%   and returns information about how many and what kind of buoys are
%   present.
%
% Input
%   blob_count = integer number of blobs in image
%   blob_hues = Nx1 vector of hues of blobs in image
%   blob_centroids = Nx2 matrix of x-y pairs of blob centroid locations
%   blob_eccentricity = Nx1 vector of blob eccentricites
%   blob_extent = Nx1 vector of blob extents
%
%   Buoy_Count_Min = integer; minimum number of buoys searched for in an
%     image (mission/controls needs requires this option)
%   Buoy_Count_Max = maximum number of buoys allowed per image; arbitrary
%     limit
%   Min_Hue,Max_Hue = Nx1 limits on valid buoy hues; hue is between 0 and 1
%   Min_Eccent,Max_Eccent = scalar limits on buoy eccentricity
%   Min_Extent,Max_Extent = scalar limits on buoy extent
%
% Output
%   successive_valid_image_count = integer value of the number of times an
%     image with more than Min_Num_Buoys is processed; persistant between
%     function calls, so that the number of successive images containing
%     at least Min_Num_Buoys buoys is tracked
%   buoy_count = integer number of buoys in image
%   buoy_hues = Nx1 vector of buoy colors
%   buoy_centroids = Nx2 matrix of x-y pairs of buoy centroid locations


% Initialize
%persistent successive_valid_image_count;
buoy_count = double(0);

%debug
%successive_valid_image_count = 0;
Buoy_Count_Max = 50;


%/debug
buoy_hues = double(zeros(Buoy_Count_Max,1));
buoy_centroids = double(-500.*ones(Buoy_Count_Max,2));  % Initialize to points clearly not located in image

buoy_id = double(-1.*ones(Buoy_Count_Max,1));
Buoy_Hue_HalfRange = 10;
Buoy1_Hue = 30;
Buoy2_Hue = 80;
Buoy3_Hue = 15;

% Loop through blobs, and analyze and extract buoy information
for i = 1:blob_count
    
    % Convert Lab to XYZ
%    R = buoy_hues(i);
%    G = buoy_hues(i);
%    B = buoy_hues(i);
    
    L = blob_hues(:,1); %refcolors(LabelMatrix(1,1,1));
    a = blob_hues(:,2);
    b = blob_hues(:,3);
    
    var_Y = L./10;
    var_X = ( a./17.5 ).*( L./10 );
    var_Z = ( b./7 ).*( L./10 );
    
    Y = var_Y.^2;
    X = ( var_X + Y )./1.02;
    Z = -( var_Z - Y )./0.847;
    
    % Convert XYZ to RGB
    var_X = X./100;        %X from 0 to  95.047      (Observer = 2 degrees, Illuminant = D65)
    var_Y = Y./100;        %Y from 0 to 100.000
    var_Z = Z./100;        %Z from 0 to 108.883
    
    var_R = var_X.*3.2406 + var_Y.*(-1.5372) + var_Z.* -0.4986;
    var_G = var_X .* -0.9689 + var_Y .*  1.8758 + var_Z.*  0.0415;
    var_B = var_X .*  0.0557 + var_Y .* -0.2040 + var_Z .*  1.0570;
    
    var_R = ( var_R > 0.0031308 ).*( 1.055.*( var_R.^( 1./2.4 ) ) - 0.055 ) + ( var_R <= 0.0031308 ).*(12.92.*var_R);
    var_G = ( var_G > 0.0031308 ).*( 1.055.*( var_G.^( 1./2.4 ) ) - 0.055 ) + ( var_G <= 0.0031308 ).*( var_G <= 12.92.*var_G );
    var_B = ( var_B > 0.0031308 ).*( 1.055 .* ( var_B .^ ( 1 ./ 2.4 ) ) - 0.055 ) + ( var_B <= 0.0031308 ).*( 12.92 .* var_B );
    
    R = var_R .* 255;
    G = var_G .* 255;
    B = var_B .* 255;
    
    % Convert RGB to HSV
    var_R = ( R ./ 255 );  % RGB from 0 to 255
    var_G = ( G ./ 255 );
    var_B = ( B ./ 255 );
    
    var_Min = min( [var_R, var_G, var_B], [], 2 );  % Min. value of RGB
    var_Max = max( [var_R, var_G, var_B], [], 2 );  % Max. value of RGB
    del_Max = var_Max - var_Min;  % Delta RGB value
    
    V = var_Max;
    
%    H = (del_Max != 0).*(  );
%    S = (del_Max != 0).*( del_Max./var_Max );
    if ( max(abs(del_Max == 0)) );  % This is a gray, no chroma...
        H = zeros(size(var_R));  % HSV results from 0 to 1
        S = zeros(size(var_R));
    else  % Chromatic data...
        
        S = del_Max ./ var_Max;
        
        del_R = ( ( ( var_Max - var_R ) ./ 6 ) + ( del_Max ./ 2 ) ) ./ del_Max;
        del_G = ( ( ( var_Max - var_G ) ./ 6 ) + ( del_Max ./ 2 ) ) ./ del_Max;
        del_B = ( ( ( var_Max - var_B ) ./ 6 ) + ( del_Max ./ 2 ) ) ./ del_Max;
        
        
        H = ( var_R == var_Max ).*( del_B - del_G ) + ( var_G == var_Max ).*( ( 1 ./ 3 ) + del_R - del_B ) + ( var_B == var_Max ).*( ( 2 ./ 3 ) + del_G - del_R );
        H = ( H < 0 ).*( H + 1 ) + ( H > 1 ).*( H - 1 );
        
        
%{        
        if( var_R == var_Max )
            H = del_B - del_G;
        elseif( var_G == var_Max )
            H = ( 1 ./ 3 ) + del_R - del_B;
        elseif( var_B == var_Max )
            H = ( 2 ./ 3 ) + del_G - del_R;
        else
            H = 0;
        end
        
        if( H < 0 )
            H = H + 1;
        end
        if( H > 1 )
            H = H - 1;
        end
%}        
    end
    
    
    
    
    
    
    
    
    
    % Store buoy information if blob conditions are met
    %   Conditions: 1) Blob eccentricity is within specified range
    %               2) Blob extent is within specified range
    %               3) Blob hue is within specified range for several buoy
    %                 types
    if( (blob_eccentricity(i)>=Min_Eccent) && (blob_eccentricity(i)<=Max_Eccent) && (blob_extent(i)>=Min_Extent) && (blob_extent(i)<=Max_Extent) )
        
        %if( (blob_hues(i)>=Buoy1_Hue-Buoy_Hue_HalfRange) && (blob_hues(i)<=Buoy1_Hue+Buoy_Hue_HalfRange) )
            buoy_count = buoy_count + 1;
            buoy_hues(buoy_count) = blob_hues(i);
            buoy_id(buoy_count) = 1;
            buoy_centroids(buoy_count,1) = blob_centroids(i,1);
            buoy_centroids(buoy_count,2) = blob_centroids(i,2);
        %end
        if( (blob_hues(i)>=Buoy2_Hue-Buoy_Hue_HalfRange) && (blob_hues(i)<=Buoy2_Hue+Buoy_Hue_HalfRange) )
            buoy_count = buoy_count + 1;
            buoy_hues(buoy_count) = blob_hues(i);
            buoy_id(buoy_count) = 2;
            buoy_centroids(buoy_count,1) = blob_centroids(i,1);
            buoy_centroids(buoy_count,2) = blob_centroids(i,2);
        end
        if( (blob_hues(i)>=Buoy3_Hue-Buoy_Hue_HalfRange) && (blob_hues(i)<=Buoy3_Hue+Buoy_Hue_HalfRange) )
            buoy_count = buoy_count + 1;
            buoy_hues(buoy_count) = blob_hues(i);
            buoy_id(buoy_count) = 3;
            buoy_centroids(buoy_count,1) = blob_centroids(i,1);
            buoy_centroids(buoy_count,2) = blob_centroids(i,2);
        end
    end
    
end

if( buoy_count >= Buoy_Count_Min )
    successive_valid_image_count_out = double(successive_valid_image_count_in + 1);
else
    successive_valid_image_count_out = double(0);
end


% Resize output arrays
%buoy_hues = buoy_hues(1:buoy_count);
%buoy_centroids = buoy_centroids(1:buoy_count,:);
%buoy_id = ;

return

== matlab function Look for Buoys/Blob Extraction ==
  data: blob_count output double; blob_hues output double; blob_centroids output double; LabelMatrix input double; ref_colors input double; blob_eccentricity output double; num_colors input double; blob_extent output double
function [blob_count, blob_hues, blob_centroids, blob_eccentricity, blob_extent] = GetBlobInfo(LabelMatrix, ref_colors, num_colors)
% This function will determine the characteristics of the blobs in an image
% given a label matrix defining the different binary images contained in a
% that label matrix
%
% Input
%   LabelMatrix = 2-D matrix of integer values, each of which represents a
%     color; location in matrix corresponds to pixel location in image
%   num_colors = integer number of colors present in LabelMatrix
%
% Output
%   blob_count = integer number of blobs in image
%   blob_hues = Nx1 vector of hues of blobs in image
%   blob_centroids = Nx2 matrix of x-y pairs of blob centroid locations
%   blob_eccentricity = Nx1 vector of blob eccentricites
%   blob_extent = Nx1 vector of blob extents


% Initialize
[rows, cols] = size(LabelMatrix);
LogicMatrix = false(rows,cols);

max_num_blobs = 50;
min_blob_area = 5;

blob_hues = double(zeros(max_num_blobs,3));
blob_centroids = double(zeros(max_num_blobs,2));
blob_eccentricity = double(zeros(max_num_blobs,1));
blob_extent = double(zeros(max_num_blobs,1));

blob_count = double(0);%uint8(0);

% Input hblob, a matrix containing [Area, blob_centroids, Eccentricity] for each
% identified blob
persistent hblob
if isempty(hblob)
    hblob = video.BlobAnalysis('AreaOutputPort',false,'BoundingBoxOutputPort',false,...
        'CentroidOutputPort',true,'EccentricityOutputPort',true,'ExtentOutputPort',true,...
        'NumBlobsOutputPort',true,'MinimumBlobAreaSource','Property',...
        'MinimumBlobArea', min_blob_area);
end

%% Calculate geometric information about the blobs
%
% LogicMatrix is a binary version of LabelMatrix, with ones at all
%   locations for which color values are k, and zeros everywhere else
for k = 1:num_colors
    for i = 1:rows
        for j = 1:cols
            if(LabelMatrix(i,j) ~= k)
                LogicMatrix(i,j) = false;
            else
                LogicMatrix(i,j) = true;
            end
        end
    end
    [TCentroid,TEccent,TExtent,TNumBlobs] = step(hblob,LogicMatrix);
    
    if(blob_count+TNumBlobs < max_num_blobs)
        for i = 1:TNumBlobs
            
            blob_centroids(blob_count+i,1) = TCentroid(1,i);
            blob_centroids(blob_count+i,2) = TCentroid(2,i);
            blob_eccentricity(blob_count+i) = TEccent(i);
            blob_extent(blob_count+i) = TExtent(i);
            
            ii = round(blob_centroids(blob_count+i,1));
            jj = round(blob_centroids(blob_count+i,2));
            blob_hues(blob_count+i,1) = ref_colors( LabelMatrix(ii,jj) );
            
        end
        blob_count = blob_count + 1;%TNumBlobs;
    end
end

return

== matlab function IterativeSegmentation/Embedded MATLAB Function1 ==
  data: R input double; RGB output double; G input double; B input double
function RGB = SeparatetoSingleSignals(R,G,B)
% This function combines the separate color signals into a single 3-D signal

[rows, cols] = size(R);

RGB = zeros(rows,cols,3);

for i = 1:rows
    for j = 1:cols
        RGB(i,j,1) = R(i,j);
        RGB(i,j,2) = G(i,j);
        RGB(i,j,3) = B(i,j);
    end
end

return
